simulink model "Lab_0_real"  (R2025b)
settings: Solver=ode4  StartTime=0.0  StopTime=20  FixedStep=.01  RelTol=1e-3
settings Model: Creator=ASUS  LastModifiedBy=ASUS

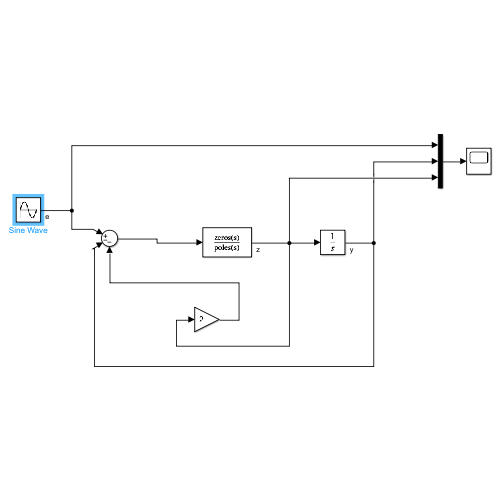
[thumbnail: Simulink's stored preview of the top-level diagram]
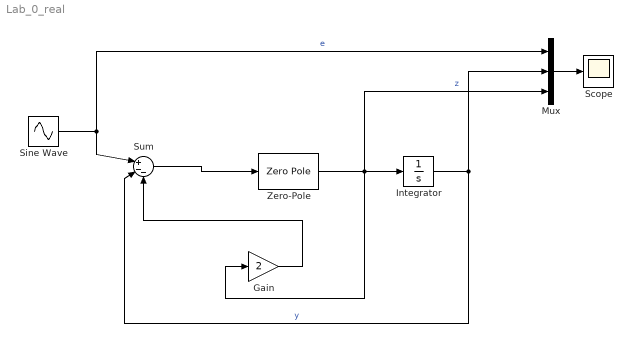
== system Lab_0_real ==
  Gain : Gain  Gain=2
  Integrator : Integrator
  Mux : Mux  Inputs=3
  Scope : Scope
  Sine Wave : Sin  Amplitude=.1  Bias=1  Frequency=5  Phase=pi/2  SampleTime=0
  Sum : Sum  Inputs=|+--
  Zero-Pole : ZeroPole  Zeros=[-5]  Poles=[0 -10]  Gain=[2]
  wires:
  Sine Wave/1 -> Sum/1, Mux/1  "e"
  Sum/1 -> Zero-Pole/1
  Gain/1 -> Sum/3
  Mux/1 -> Scope/1
  Integrator/1 -> Mux/2, Sum/2  "y"
  Zero-Pole/1 -> Gain/1, Mux/3, Integrator/1  "z"
